simulink model "sampleModel1483"  (R2023a)
settings: Solver=VariableStepAuto  StartTime=0.0  StopTime=10.0  RelTol=1e-3
libraries: hdlsllib x6, simulink x1
settings Model: Creator=user1  LastModifiedBy=user1

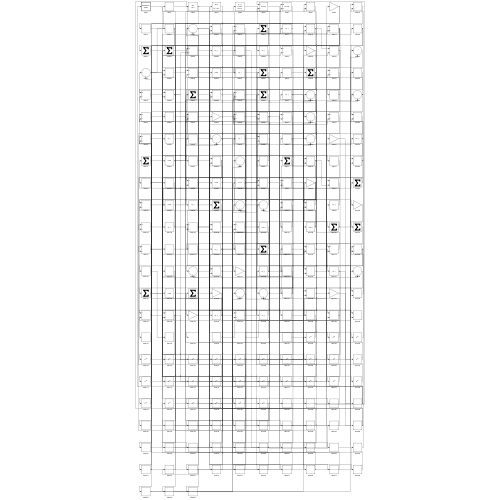
[thumbnail: Simulink's stored preview of the top-level diagram]
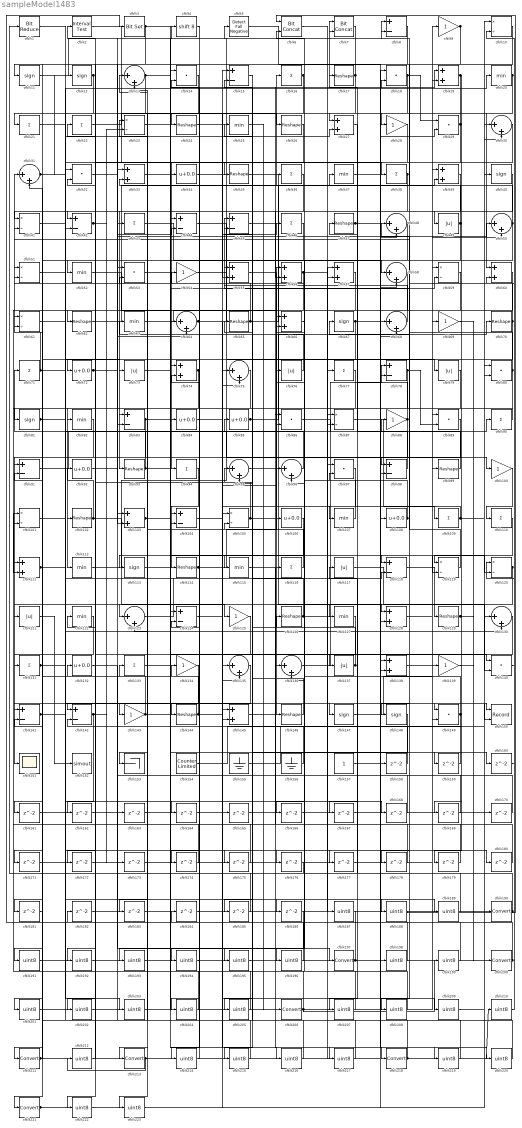
== system sampleModel1483 ==
  cfblk1 : hdlsllib/Logic and Bit Operations/Bit Reduce  mode=AND
  cfblk{10,23,41,51,59,61,87,101,105,119..120} (11 alike) : Product  Inputs=*/  RndMeth=Zero  SaturateOnIntegerOverflow=on
  cfblk{9,28,54,69,88,100,125,134,139,143} (10 alike) : Gain
  cfblk{17,24,26,35,47,62,65,70,93,99,102,114,126,129,144,146} (16 alike) : Reshape
  cfblk{19,27,33,39,55..57,60,66,74,103,111,128,138,145} (15 alike) : Sum
  cfblk{8,15,42,44..45,78,83,91,98,104,118,124,141..142} (14 alike) : Sum  Inputs=+-
  cfblk{34,72,84..85,92,106,108,132} (8 alike) : Bias  Bias=0.0  SaturateOnIntegerOverflow=off
  cfblk{20,25,37,52,63,82,107,112,115,122,127} (11 alike) : MinMax
  cfblk{16,21..22,36,38,43,46,71,77,90,94,109..110,116,131,133} (16 alike) : Sum  Inputs=+
  cfblk{11..12,40,67,81,113,147..148} (8 alike) : Signum
  cfblk{49,73,76,79,117,121,137} (7 alike) : Abs  SaturateOnIntegerOverflow=off
  cfblk{13,30..31,48,50,58,64,68,75,95..96,123,130,135..136} (15 alike) : Sum  Inputs=|++
  cfblk{14,18,29,32,53,80,86,89,97,140,149} (11 alike) : DotProduct  OutDataTypeStr=Inherit: Inherit via internal rule
  cfblk150 : Record  FileSettingsInternal="{\"entries\":[{\"content\":{\"excelSettings\":{\"content\":{},\"type\":\"Streamout.ExcelSettings\"}},\"type\":\"Streamout.FileSettingStorage\",\"uuid\":\"\"}],\"packageUris\":[\"http:\\/\\/schema.mathworks.com\\/mf0\\/streamout_blocks\\/R2020a\"],\"version\":\"1.0\"}"  Layout=[1 1]  SignalsInternal="{\"entries\":[{\"content\":{\"signals\":[{\"content\":{\"blockPath\":[],\"dimensions\":[1],\"domain\":\"\",\"lineColor\":\"#a2142f\",\"plots\":[1],\"port\":1,\"signalID\":1100,\"signalName\":\"XY Graph:1\"},\"type\":\"RecordBlkView.Signal\",\"uuid\":\"\"},{\"content\":{\"blockPath\":[],\"dimensions\":[1],\"domain\":\"\",\"lineColor\":\"#139fff\",\"plots\":[1],\"port\":2,\"signalID\":1103,\"signalName\":\"XY Graph:2\"},\"type\":\"RecordBlkView.Signal\",\"uuid\":\"\"}]},\"type\":\"RecordBlkView.InputSignals\",\"uuid\":\"\"}],\"packageUris\":[\"http:\\/\\/schema.mathworks.com\\/mf0\\/streamout_blocks\\/R2020a\"],\"version\":\"1.0\"}"  VisualizationBindings="{\"xyplotplugin\":{\"info\":[{\"series\":[{\"bindingParametersList\":[{\"parameter\":\"X-Axis\",\"signalID\":1100,\"signalName\":\"XY Graph:1\"},{\"parameter\":\"Y-Axis\",\"signalID\":1103,\"signalName\":\"XY Graph:2\"}],\"seriesID\":10004}],\"subplotID\":1}]}}"  CompatibilityTag=XY  st=-1
  cfblk151 : Scope
  cfblk152 : ToWorkspace  VariableName=simout  SaveFormat=Timeseries  SampleTime=-1
  cfblk153 : Terminator
  cfblk154 : hdlsllib/Sources/Counter Limited  uplimit=7  tsamp=-1
  cfblk155 : Ground
  cfblk156 : Ground
  cfblk157 : Constant  SampleTime=-1
  cfblk{158..186} (29 alike) : Delay  SampleTime=1
  cfblk{187..189,191..196,198..199,201..205,207..210,212,214..217,219..220,222..223} (29 alike) : DataTypeConversion  OutDataTypeStr=uint8  SaturateOnIntegerOverflow=off  RndMeth=Floor
  cfblk{190,197,200,206,211,213,218,221} (8 alike) : DataTypeConversion  SaturateOnIntegerOverflow=off  RndMeth=Floor
  cfblk2 : hdlsllib/Logic and Bit Operations/Interval Test  IntervalClosedRight=on  uplimit=0.5  IntervalClosedLeft=on  lowlimit=-0.5  OutDataTypeStr=boolean
  cfblk3 : simulink/Logic and Bit Operations/Bit Set  iBit=0
      settings: LibrarySourceBlock=|
      | hdlsllib/Logic and Bit
      | Operations/Bit Set
  cfblk4 : ArithShift  BitShiftNumber=8
  cfblk5 : hdlsllib/Logic and Bit Operations/Detect Fall Negative  vinit=0  OutDataTypeStr=boolean
  cfblk6 : hdlsllib/Logic and Bit Operations/Bit Concat  numInputs=2
  cfblk7 : hdlsllib/Logic and Bit Operations/Bit Concat  numInputs=2
  wires:
  cfblk22/1 -> cfblk24/1
  cfblk40/1 -> cfblk93/1
  cfblk126/1 -> cfblk128/1, cfblk95/1, cfblk96/2
  cfblk87/1 -> cfblk109/1
  cfblk58/1 -> cfblk146/1
  cfblk64/1 -> cfblk8/1, cfblk150/1
  cfblk136/1 -> cfblk78/1
  cfblk82/1 -> cfblk151/1
  cfblk94/1 -> cfblk114/1
  cfblk99/1 -> cfblk67/1
  cfblk74/1 -> cfblk113/1, cfblk193/1
  cfblk80/1 -> cfblk112/1, cfblk55/1
  cfblk69/1 -> cfblk190/1
  cfblk38/1 -> cfblk41/1, cfblk167/1
  cfblk65/1 -> cfblk37/1, cfblk51/1
  cfblk2/1 -> cfblk87/1
  cfblk62/1 -> cfblk16/1
  cfblk60/1 -> cfblk137/1
  cfblk28/1 -> cfblk94/1
  cfblk44/1 -> cfblk100/1
  cfblk68/1 -> cfblk45/1
  cfblk76/1 -> cfblk63/1
  cfblk4/1 -> cfblk144/1
  cfblk54/1 -> cfblk79/1
  cfblk20/1 -> cfblk60/1, cfblk148/1
  cfblk83/1 -> cfblk102/1, cfblk118/1
  cfblk12/1 -> cfblk141/1, cfblk201/1
  cfblk133/1 -> cfblk74/1
  cfblk32/1 -> cfblk4/1
  cfblk35/1 -> cfblk127/1
  cfblk30/1 -> cfblk72/1
  cfblk96/1 -> cfblk71/1
  cfblk139/1 -> cfblk200/1
  cfblk90/1 -> cfblk84/1
  cfblk102/1 -> cfblk125/1, cfblk92/1
  cfblk71/1 -> cfblk31/1, cfblk150/2
  cfblk3/1 -> cfblk26/1, cfblk83/2
  cfblk122/1 -> cfblk211/1
  cfblk92/1 -> cfblk50/1
  cfblk31/1 -> cfblk12/1, cfblk176/1, cfblk177/1
  cfblk121/1 -> cfblk152/1
  cfblk101/1 -> cfblk20/1
  cfblk86/1 -> cfblk90/1
  cfblk140/1 -> cfblk120/1
  cfblk34/1 -> cfblk38/1
  cfblk81/1 -> cfblk86/2, cfblk175/1
  cfblk104/1 -> cfblk46/1
  cfblk109/1 -> cfblk107/1, cfblk30/2
  cfblk135/1 -> cfblk221/1
  cfblk78/1 -> cfblk89/2, cfblk166/1
  cfblk113/1 -> cfblk140/1
  cfblk55/1 -> cfblk136/1
  cfblk23/1 -> cfblk147/1
  cfblk114/1 -> cfblk56/1, cfblk96/1
  cfblk112/1 -> cfblk88/1
  cfblk119/1 -> cfblk48/1
  cfblk103/1 -> cfblk59/2, cfblk159/1
  cfblk95/1 -> cfblk120/2
  cfblk142/1 -> cfblk162/1, cfblk163/1
  cfblk63/1 -> cfblk66/1
  cfblk138/1 -> cfblk99/1
  cfblk85/1 -> cfblk70/1, cfblk19/1
  cfblk108/1 -> cfblk97/2, cfblk51/2
  cfblk120/1 -> cfblk121/1, cfblk136/2
  cfblk25/1 -> cfblk206/1
  cfblk5/1 -> cfblk128/2
  cfblk56/1 -> cfblk160/1, cfblk161/1
  cfblk57/1 -> cfblk111/2
  cfblk137/1 -> cfblk36/1, cfblk105/2
  cfblk36/1 -> cfblk56/2
  cfblk98/1 -> cfblk47/1
  cfblk11/1 -> cfblk5/1
  cfblk134/1 -> cfblk213/1
  cfblk145/1 -> cfblk39/2
  cfblk146/1 -> cfblk65/1
  cfblk24/1 -> cfblk7/1
  cfblk143/1 -> cfblk22/1, cfblk7/2
  cfblk18/1 -> cfblk82/1, cfblk29/1
  cfblk73/1 -> cfblk34/1
  cfblk97/1 -> cfblk145/2
  cfblk117/1 -> cfblk140/2
  cfblk67/1 -> cfblk29/2, cfblk191/1
  cfblk88/1 -> cfblk138/2, cfblk104/2, cfblk153/1, cfblk17/1, cfblk91/1
  cfblk93/1 -> cfblk149/1, cfblk32/2
  cfblk39/1 -> cfblk123/1
  cfblk47/1 -> cfblk68/1, cfblk119/2
  cfblk129/1 -> cfblk169/1, cfblk170/1
  cfblk118/1 -> cfblk129/1
  cfblk48/1 -> cfblk116/1, cfblk52/1
  cfblk42/1 -> cfblk23/2, cfblk172/1, cfblk173/1
  cfblk123/1 -> cfblk48/2
  cfblk111/1 -> cfblk130/2, cfblk27/2
  cfblk131/1 -> cfblk118/2, cfblk168/1
  cfblk105/1 -> cfblk2/1, cfblk106/1
  cfblk89/1 -> cfblk143/1
  cfblk52/1 -> cfblk64/1
  cfblk124/1 -> cfblk197/1
  cfblk107/1 -> cfblk85/1
  cfblk100/1 -> cfblk110/1
  cfblk13/1 -> cfblk103/2, cfblk186/1, cfblk220/1
  cfblk33/1 -> cfblk18/2
  cfblk70/1 -> cfblk142/1, cfblk41/2
  cfblk116/1 -> cfblk13/2
  cfblk144/1 -> cfblk75/2, cfblk91/2
  cfblk91/1 -> cfblk43/1
  cfblk59/1 -> cfblk115/1
  cfblk17/1 -> cfblk11/1, cfblk42/2
  cfblk50/1 -> cfblk78/2, cfblk23/1
  cfblk43/1 -> cfblk58/1
  cfblk149/1 -> cfblk76/1, cfblk142/2
  cfblk128/1 -> cfblk50/2
  cfblk156/1 -> cfblk74/2
  cfblk141/1 -> cfblk61/1, cfblk180/1
  cfblk21/1 -> cfblk73/1
  cfblk16/1 -> cfblk95/2, cfblk171/1
  cfblk53/1 -> cfblk218/1
  cfblk154/1 -> cfblk58/2
  cfblk1/1 -> cfblk35/1
  cfblk75/1 -> cfblk101/2
  cfblk29/1 -> cfblk98/1, cfblk28/1, cfblk119/1
  cfblk72/1 -> cfblk64/2, cfblk44/2
  cfblk9/1 -> cfblk131/1, cfblk62/1
  cfblk49/1 -> cfblk8/2, cfblk174/1
  cfblk155/1 -> cfblk30/1
  cfblk45/1 -> cfblk57/2
  cfblk8/1 -> cfblk42/1
  cfblk147/1 -> cfblk9/1
  cfblk7/1 -> cfblk21/1
  cfblk19/1 -> cfblk83/1, cfblk49/1, cfblk55/2, cfblk81/1, cfblk27/1
  cfblk158/1 -> cfblk45/2
  cfblk159/1 -> cfblk57/1
  cfblk160/1 -> cfblk60/2
  cfblk161/1 -> cfblk68/2
  cfblk162/1 -> cfblk39/1
  cfblk163/1 -> cfblk33/2
  cfblk41/1 -> cfblk164/1
  cfblk165/1 -> cfblk18/1
  cfblk166/1 -> cfblk138/1
  cfblk167/1 -> cfblk130/1
  cfblk168/1 -> cfblk103/1
  cfblk169/1 -> cfblk13/1
  cfblk170/1 -> cfblk59/1
  cfblk171/1 -> cfblk149/2
  cfblk172/1 -> cfblk87/2
  cfblk173/1 -> cfblk98/2
  cfblk174/1 -> cfblk123/2
  cfblk175/1 -> cfblk105/1
  cfblk176/1 -> cfblk1/1
  cfblk177/1 -> cfblk19/2
  cfblk79/1 -> cfblk178/1
  cfblk178/1 -> cfblk101/1
  cfblk110/1 -> cfblk179/1
  cfblk179/1 -> cfblk86/1
  cfblk180/1 -> cfblk66/2
  cfblk46/1 -> cfblk181/1
  cfblk181/1 -> cfblk31/2
  cfblk182/1 -> cfblk80/2
  cfblk106/1 -> cfblk183/1
  cfblk183/1 -> cfblk75/1
  cfblk26/1 -> cfblk185/1
  cfblk185/1 -> cfblk145/1
  cfblk6/1 -> cfblk187/1
  cfblk187/1 -> cfblk3/1
  cfblk51/1 -> cfblk188/1
  cfblk188/1 -> cfblk6/1
  cfblk157/1 -> cfblk189/1
  cfblk189/1 -> cfblk6/2
  cfblk190/1 -> cfblk89/1, cfblk117/1, cfblk33/1
  cfblk191/1 -> cfblk69/1
  cfblk14/1 -> cfblk192/1
  cfblk192/1 -> cfblk165/1
  cfblk193/1 -> cfblk14/1
  cfblk125/1 -> cfblk194/1
  cfblk194/1 -> cfblk14/2
  cfblk132/1 -> cfblk195/1
  cfblk195/1 -> cfblk80/1
  cfblk66/1 -> cfblk196/1
  cfblk196/1 -> cfblk132/1
  cfblk197/1 -> cfblk133/1, cfblk219/1
  cfblk37/1 -> cfblk198/1
  cfblk198/1 -> cfblk124/1
  cfblk199/1 -> cfblk124/2
  cfblk200/1 -> cfblk44/1, cfblk54/1
  cfblk201/1 -> cfblk139/1
  cfblk77/1 -> cfblk202/1
  cfblk202/1 -> cfblk104/1
  cfblk61/1 -> cfblk203/1
  cfblk203/1 -> cfblk77/1
  cfblk184/1 -> cfblk204/1
  cfblk204/1 -> cfblk111/1
  cfblk148/1 -> cfblk205/1
  cfblk205/1 -> cfblk184/1
  cfblk206/1 -> cfblk199/1, cfblk182/1
  cfblk27/1 -> cfblk207/1
  cfblk207/1 -> cfblk25/1
  cfblk10/1 -> cfblk208/1
  cfblk208/1 -> cfblk126/1
  cfblk84/1 -> cfblk209/1
  cfblk209/1 -> cfblk10/1
  cfblk210/1 -> cfblk10/2
  cfblk211/1 -> cfblk61/2, cfblk97/1
  cfblk212/1 -> cfblk122/1
  cfblk213/1 -> cfblk212/1, cfblk158/1
  cfblk130/1 -> cfblk214/1
  cfblk214/1 -> cfblk134/1
  cfblk15/1 -> cfblk215/1
  cfblk215/1 -> cfblk32/1
  cfblk164/1 -> cfblk216/1
  cfblk216/1 -> cfblk15/1
  cfblk115/1 -> cfblk217/1
  cfblk217/1 -> cfblk15/2
  cfblk218/1 -> cfblk210/1, cfblk141/2
  cfblk219/1 -> cfblk53/1
  cfblk220/1 -> cfblk53/2
  cfblk221/1 -> cfblk108/1, cfblk40/1
  cfblk127/1 -> cfblk222/1
  cfblk222/1 -> cfblk135/1
  cfblk186/1 -> cfblk223/1
  cfblk223/1 -> cfblk135/2
